simulink model "control"  (R2020a)
settings: Solver=FixedStepAuto  StartTime=0.0  StopTime=sim_duration  FixedStep=time_step  RelTol=1e-3
values from neighbouring files (symbols this model uses):
  duty_init = 0.5    [control_script.m]
  Voc = num_cells_series * Voc_per_cell    (= 21.6)    [control_script.m]
libraries: nesl_utility x5, fl_lib x4, ee_lib x3, simulink x2
settings Model: Creator=HP  LastModifiedBy=HP

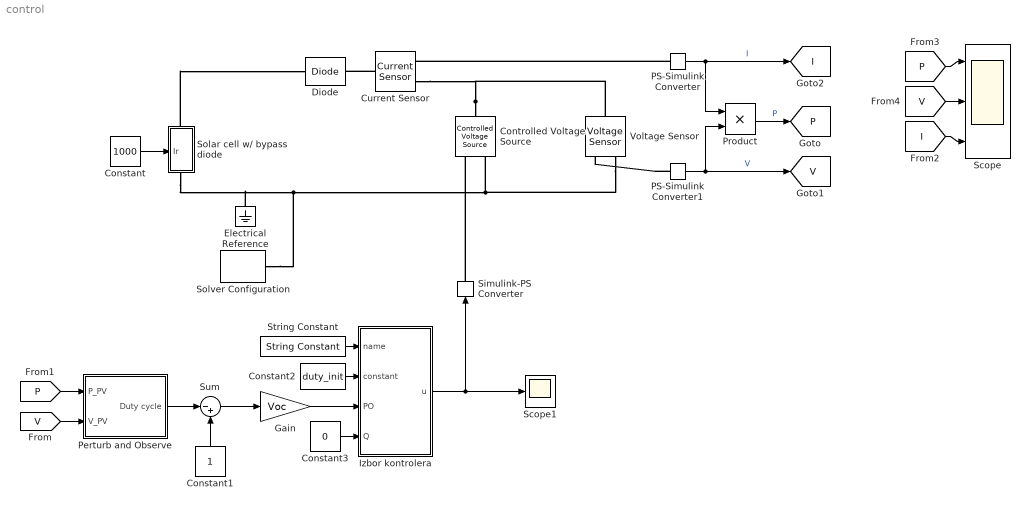
== system control ==
  Constant : Constant  Value=1000
  Constant1 : Constant
  Constant2 : Constant  Value=duty_init
  Constant3 : Constant  Value=0
  Controlled Voltage Source : fl_lib/Electrical/Electrical Sources/Controlled Voltage Source
  Current Sensor : fl_lib/Electrical/Electrical Sensors/Current Sensor
  Diode : ee_lib/Semiconductors & Converters/Diode  ModelType=ee.enum.diode.modelType.pwl  Vf=0.1 V  Ron=0.01 Ohm  Goff=1e-8 S  prmExp=ee.enum.diode.expParam.useTwo  I12=[.0137, .545] A  V12=[.6, .7] V  IS=1e-12 A  ec=1  I1=0.0137 A  V1=0.6 V  RS=0 Ohm  Tmeas=25 degC  N_series=1  N_parallel=1  Rz=0.3 Ohm  BV=inf V  C_param=ee.enum.diode.capParam.fixed  CJ=0 pF  CJ0=5 pF  VJ=1 V  Mgrad=0.5  Vvec=[.1, 10, 100] V  Cvec=[3.5, 1, .4] pF  FC=0.5  Q_param=ee.enum.diode.recoveryParam.off  iRM=-7.15 A  iF=4 A  didt=-750 A/us  trr_factor=3  trr=115 ns  Qrr=1500 s*uA  TT=50 ns  tau=100 ns  T_param=ee.enum.diode.temperatureParam.off  IS_T2=1.25e-7 A  I1_T2=0.245 A  V1_T2=0.5 V  Tmeas2=125 degC  EG_param=ee.enum.diode.egapParam.material_si  EG=1.11 eV  XTI_param=ee.enum.diode.xtiParam.pn  XTI=3  dBVdT=0 V/K  Tdevice=25 degC  i_specify=off  i_priority=None  i=0 A  i_nominal_specify=off  i_nominal_unit=A  i_nominal_value=1  v_specify=off  v_priority=None  v=0 V  v_nominal_specify=off  v_nominal_unit=V  v_nominal_value=1  i_capacitor_specify=off  i_capacitor_priority=None  i_capacitor=0 A  i_capacitor_nominal_specify=off  i_capacitor_nominal_unit=A  i_capacitor_nominal_value=1  v_capacitor_specify=off  v_capacitor_priority=None  v_capacitor=0 V  v_capacitor_nominal_specify=off  v_capacitor_nominal_unit=V  v_capacitor_nominal_value=1  power_dissipated_specify=off  power_dissipated_priority=None  power_dissipated=0 W  power_dissipated_nominal_specify=off  power_dissipated_nominal_unit=W  power_dissipated_nominal_value=1  thermal_network_parameterization=ee.enum.thermalNetworkTopology.cauer  Rth=[0, 10] K/W  Rth_Foster=[4, 6] K/W  thermal_mass_parameterization=ee.enum.thermalNetwork.timeconstant  thermal_mass=[0, 1] J/K  thermal_mass_Foster=[1.5, 3] J/K  thermal_time_constant=[0, 10] s  thermal_time_constant_Foster=[6, 18] s  thermal_mass_initial_temperatures=[25, 25] degC
  Electrical Reference : fl_lib/Electrical/Electrical Elements/Electrical Reference
  Gain : Gain  Gain=Voc
  Izbor kontrolera : Subsystem
  PS-Simulink Converter : nesl_utility/PS-Simulink Converter  PhysicalDomain=network_engine_domain  SubClassName=ps_output  LeftPortType=input  RightPortType=output  PseudoPeriodic=off  Frequencies=[]  Unit=inherit  AffineConversion=off
  PS-Simulink Converter1 : nesl_utility/PS-Simulink Converter  PhysicalDomain=network_engine_domain  SubClassName=ps_output  LeftPortType=input  RightPortType=output  PseudoPeriodic=off  Frequencies=[]  Unit=inherit  AffineConversion=off
  Perturb and Observe : Subsystem
  Product : Product
  Scope : Scope  NumInputPorts=3
  Scope1 : Scope
  Simulink-PS Converter : nesl_utility/Simulink-PS Converter  PhysicalDomain=network_engine_domain  SubClassName=ps_input  LeftPortType=input  RightPortType=output  PseudoPeriodic=off  Frequencies=[]  NoiseDistribution=none  NoiseParameters=[]  Unit=1  AffineConversion=off  FilteringAndDerivatives=provide  SimscapeFilterOrder=1  InputFilterTimeConstant=0.001  UdotUserProvided=0
  Solar cell w/ bypass diode : Subsystem
      settings: PortSchema="{\"entries\":[{\"content\":{\"sides\":[{\"content\":{\"connectorIds\":[\"LConn1\"]},\"type\":\"ConnectorPlacement.EquallySpacedRectSide\",\"uuid\":\"9ae7f0a8-84a6-4a03-968b-1625bd6cfd8b\"},{\"content\":{\"connectorIds\":[\"RConn1\"],\"side\":\"RIGHT\"},\"type\":\"ConnectorPlacement.EquallySpacedRectSide\",\"uuid\":\"f022b796-d1b7-473b-900e-02078c66088c\"},{\"content\":{\"connectorIds\":[\"In1\"],\"side\":\"TOP\"},\"type\":\"ConnectorPlacement.EquallySpacedRectSide\",\"uuid\":\"3e1f2411-29ae-4e6f-a71a-fe75fbcf935f\"}]},\"type\":\"ConnectorPlacement.EquallySpacedConnector\",\"uuid\":\"ebd2d106-414a-4764-a949-46f428e99ff1\"}],\"packageUris\":[\"http://schema.mathworks.com/mf0/Connector/19700101\"],\"version\":\"1.0\"}"
  Solver Configuration : nesl_utility/Solver Configuration  PhysicalDomain=network_engine_domain  SubClassName=solver  LeftPortType=input  RightPortType=generic  Tones=[]  Harmonics=[]  SimulateNoise=off  Profile=off  UseLocalSampling=off  EnableSwitchedLinearOptims=on  FrequencyDomain=off  UseCCode=off  RelTol=0.001  AbsTol=1e-06  MinStep=1e-09  ToWorkspace=off  RevertToSquareIcSolve=off  NumHomotopyIterations=100  PhasorMode=off  PhasorModeNumHarmonics=1  DoDC=off  ResidualTolerance=1e-09  UseLocalSolver=off  LocalSolverChoice=NE_BACKWARD_EULER_ADVANCER  LocalSolverSampleTime=1e-3  DoFixedCost=off  MaxNonlinIter=3  MaxModeIter=2  LinearAlgebra=auto  EquationFormulation=NE_TIME_EF  DelaysMemoryBudget=1024  AutomaticFiltering=on  FilteringTimeConstant=0.001  PartitionStorageMethod=AS_NEEDED  PartitionMemoryBudget=1024  PartitionMethod=ROBUST
  String Constant : StringConstant  String=mppt_algo_name
  Sum : Sum  Inputs=|-+
  Voltage Sensor : fl_lib/Electrical/Electrical Sensors/Voltage Sensor
  tag scope: I=global, P=global, V=global
  wires:
  Product/1 -> [P]  "P"
  PS-Simulink Converter1/1 -> [V], Product/2  "V"
  Constant/1 -> Solar cell w/ bypass diode/1(Ir)
  PS-Simulink Converter/1 -> [I], Product/1  "I"
  Perturb and Observe/1(Duty cycle) -> Sum/1
  Sum/1 -> Gain/1
  Constant1/1 -> Sum/2
  [V] -> Perturb and Observe/2(V_PV)
  [P] -> Perturb and Observe/1(P_PV)
  Gain/1 -> Izbor kontrolera/3(PO)
  String Constant/1 -> Izbor kontrolera/1(name)
  Constant3/1 -> Izbor kontrolera/4(Q)
  Constant2/1 -> Izbor kontrolera/2(constant)
  Izbor kontrolera/1(u) -> Scope1/1, Simulink-PS Converter/1
  [I] -> Scope/3
  [P] -> Scope/1
  [V] -> Scope/2
  connections:
  Controlled Voltage Source/LConn1 -- Current Sensor/RConn2 -- Voltage Sensor/LConn1
  Voltage Sensor/RConn2 -- Controlled Voltage Source/RConn2 -- Solver Configuration/RConn1 -- Electrical Reference/LConn1 -- Solar cell w/ bypass diode/LConn1
  PS-Simulink Converter/LConn1 -- Current Sensor/RConn1
  Current Sensor/LConn1 -- Diode/RConn1
  Solar cell w/ bypass diode/RConn1 -- Diode/LConn1
  PS-Simulink Converter1/LConn1 -- Voltage Sensor/RConn1
  Simulink-PS Converter/RConn1 -- Controlled Voltage Source/RConn1

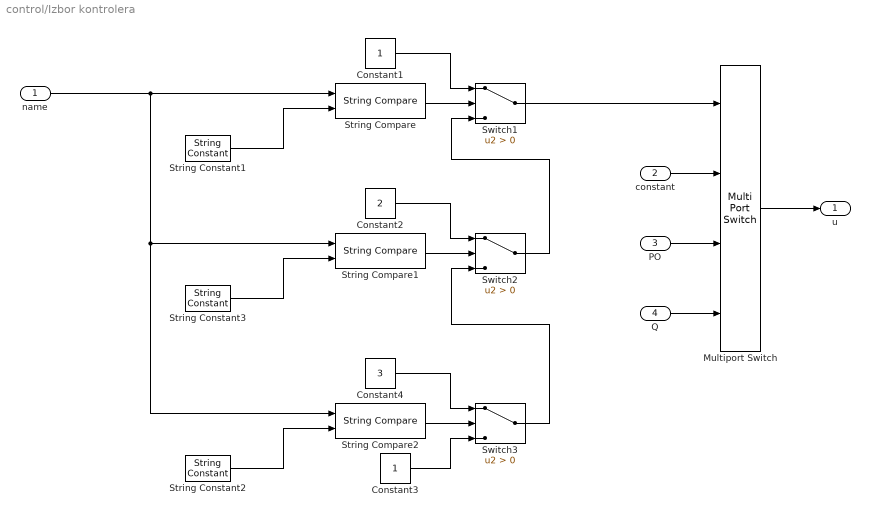
== system control/Izbor kontrolera ==
  name : Inport
  constant : Inport  Port=2
  PO : Inport  Port=3
  Q : Inport  Port=4
  Constant1 : Constant
  Constant2 : Constant  Value=2
  Constant3 : Constant
  Constant4 : Constant  Value=3
  Multiport Switch : MultiPortSwitch
  String Compare : StringCompare
  String Compare1 : StringCompare
  String Compare2 : StringCompare
  String Constant1 : StringConstant  String="\"constant\""
  String Constant2 : StringConstant  String="\"q\""
  String Constant3 : StringConstant  String="\"po\""
  Switch1 : Switch  Criteria=u2 > Threshold
  Switch2 : Switch  Criteria=u2 > Threshold
  Switch3 : Switch  Criteria=u2 > Threshold
  u : Outport
  wires:
  String Compare1/1 -> Switch2/2
  Switch1/1 -> Multiport Switch/1
  String Constant1/1 -> String Compare/2
  String Constant3/1 -> String Compare1/2
  Constant1/1 -> Switch1/1
  Constant2/1 -> Switch2/1
  Switch2/1 -> Switch1/3
  String Compare/1 -> Switch1/2
  PO/1 -> Multiport Switch/3
  Multiport Switch/1 -> u/1
  constant/1 -> Multiport Switch/2
  Q/1 -> Multiport Switch/4
  String Compare2/1 -> Switch3/2
  String Constant2/1 -> String Compare2/2
  Constant4/1 -> Switch3/1
  Switch3/1 -> Switch2/3
  name/1 -> String Compare/1, String Compare2/1, String Compare1/1
  Constant3/1 -> Switch3/3

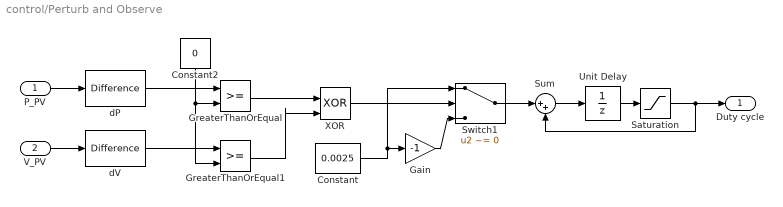
== system control/Perturb and Observe ==
  P_PV : Inport
  V_PV : Inport  Port=2
  Constant : Constant  Value=0.0025
  Constant2 : Constant  Value=0
  Gain : Gain  Gain=-1
  GreaterThanOrEqual : RelationalOperator  OutDataTypeStr=boolean  RndMeth=Simplest
  GreaterThanOrEqual1 : RelationalOperator  OutDataTypeStr=boolean  RndMeth=Simplest
  Saturation : Saturate  UpperLimit=1  LowerLimit=0
  Sum : Sum  Inputs=|++
  Switch1 : Switch  Criteria=u2 ~= 0
  Unit Delay : UnitDelay  InitialCondition=duty_init  SampleTime=-1  HasFrameUpgradeWarning=on
  XOR : Logic  Operator=XOR  IconShape=distinctive  AllPortsSameDT=off  OutDataTypeStr=boolean
  dP : simulink/Discrete/Difference  ICPrevInput=0.0  OutMin=[]  OutMax=[]  OutDataType=fixdt(1, 16)  OutScaling=2^-10  DoSatur=off
  dV : simulink/Discrete/Difference  ICPrevInput=0.0  OutMin=[]  OutMax=[]  OutDataType=fixdt(1, 16)  OutScaling=2^-10  DoSatur=off
  Duty cycle : Outport
  wires:
  Switch1/1 -> Sum/1
  Sum/1 -> Unit Delay/1
  Saturation/1 -> Duty cycle/1, Sum/2
  GreaterThanOrEqual1/1 -> XOR/2
  Constant/1 -> Switch1/1, Gain/1
  Constant2/1 -> GreaterThanOrEqual1/2, GreaterThanOrEqual/2
  dP/1 -> GreaterThanOrEqual/1
  XOR/1 -> Switch1/2
  dV/1 -> GreaterThanOrEqual1/1
  Unit Delay/1 -> Saturation/1
  GreaterThanOrEqual/1 -> XOR/1
  Gain/1 -> Switch1/3
  V_PV/1 -> dV/1
  P_PV/1 -> dP/1

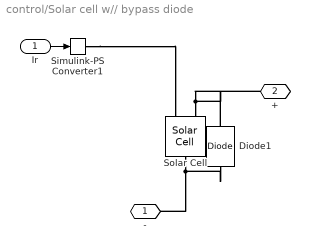
== system control/Solar cell w// bypass diode ==
  Ir : Inport
  Diode1 : ee_lib/Semiconductors & Converters/Diode  ModelType=ee.enum.diode.modelType.pwl  Vf=0.6 V  Ron=0.01 Ohm  Goff=eps S  prmExp=ee.enum.diode.expParam.useTwo  I12=[.0137, .545] A  V12=[.6, .7] V  IS=1e-12 A  ec=1  I1=0.0137 A  V1=0.6 V  RS=0 Ohm  Tmeas=25 degC  N_series=1  N_parallel=1  Rz=0.3 Ohm  BV=inf V  C_param=ee.enum.diode.capParam.fixed  CJ=0 pF  CJ0=5 pF  VJ=1 V  Mgrad=0.5  Vvec=[.1, 10, 100] V  Cvec=[3.5, 1, .4] pF  FC=0.5  Q_param=ee.enum.diode.recoveryParam.off  iRM=-7.15 A  iF=4 A  didt=-750 A/us  trr_factor=3  trr=115 ns  Qrr=1500 s*uA  TT=50 ns  tau=100 ns  T_param=ee.enum.diode.temperatureParam.off  IS_T2=1.25e-7 A  I1_T2=0.245 A  V1_T2=0.5 V  Tmeas2=125 degC  EG_param=ee.enum.diode.egapParam.material_si  EG=1.11 eV  XTI_param=ee.enum.diode.xtiParam.pn  XTI=3  dBVdT=0 V/K  Tdevice=25 degC  i_specify=off  i_priority=None  i=0 A  i_nominal_specify=off  i_nominal_unit=A  i_nominal_value=1  v_specify=off  v_priority=None  v=0 V  v_nominal_specify=off  v_nominal_unit=V  v_nominal_value=1  i_capacitor_specify=off  i_capacitor_priority=None  i_capacitor=0 A  i_capacitor_nominal_specify=off  i_capacitor_nominal_unit=A  i_capacitor_nominal_value=1  v_capacitor_specify=off  v_capacitor_priority=None  v_capacitor=0 V  v_capacitor_nominal_specify=off  v_capacitor_nominal_unit=V  v_capacitor_nominal_value=1  power_dissipated_specify=off  power_dissipated_priority=None  power_dissipated=0 W  power_dissipated_nominal_specify=off  power_dissipated_nominal_unit=W  power_dissipated_nominal_value=1  thermal_network_parameterization=ee.enum.thermalNetworkTopology.cauer  Rth=[0, 10] K/W  Rth_Foster=[4, 6] K/W  thermal_mass_parameterization=ee.enum.thermalNetwork.timeconstant  thermal_mass=[0, 1] J/K  thermal_mass_Foster=[1.5, 3] J/K  thermal_time_constant=[0, 10] s  thermal_time_constant_Foster=[6, 18] s  thermal_mass_initial_temperatures=[25, 25] degC
  Simulink-PS Converter1 : nesl_utility/Simulink-PS Converter  PhysicalDomain=network_engine_domain  SubClassName=ps_input  LeftPortType=input  RightPortType=output  PseudoPeriodic=off  Frequencies=[]  NoiseDistribution=none  NoiseParameters=[]  Unit=1  AffineConversion=off  FilteringAndDerivatives=provide  SimscapeFilterOrder=1  InputFilterTimeConstant=0.001  UdotUserProvided=0
  Solar Cell : ee_lib/Sources/Solar Cell  prm=1  Isc=Isc A  Voc=Voc_per_cell V  Is=1e-6 A  Is2=0 A  Iph=7.34 A  Ir0=1000 W/m^2  ec=1.5  N2=2  Rs=0 Ohm  Rp=inf Ohm  N_series=num_cells_series  TIPH1=0 1/K  EG=1.11 eV  TXIS1=3  TXIS2=3  TRS1=0  TRP1=0  Tmeas=25 degC  TFIXED=25 degC  thermal_mass=100 J/K  initial_temperature=25 degC
      settings: SourceProductBaseCode=PS
  - : PMIOPort  Side=Left
  + : PMIOPort  Port=2  Side=Right
  wires:
  Ir/1 -> Simulink-PS Converter1/1
  connections:
  Diode1/LConn1 -- -/RConn1 -- Solar Cell/RConn1
  Simulink-PS Converter1/RConn1 -- Solar Cell/LConn1
  Solar Cell/LConn2 -- +/RConn1 -- Diode1/RConn1
